simulink model "eovsa_corr_300mhz"  (R2012b)
settings: Solver=VariableStepDiscrete  SolverMode=SingleTasking  StartTime=0.0  StopTime=5000  RelTol=1e-3
undefined symbols (not defined in the file or in its folder): A, B, gcbh, PCIN, sfp, xlBlockLoadCallback, xlipgetpartsetting
libraries: xbsIndex_r4 x5996, casper_library_misc x52, simulink x33, dspsigops x24, xps_library x15, casper_library_delays x2
(part 25 of 65)

== system eovsa_corr_300mhz/swreg/pkt_fft ==
  sim_1 : Inport
  eovsa_corr_300mhz_swreg_pkt_fft_user_data_out : xbsIndex_r4/Gateway In  gui_display_data_type=Fixed-point  arith_type=Unsigned  n_bits=32  bin_pt=0  preci_type=Single  exp_width=8  frac_width=24  quantization="Round  (unbiased: +/- Inf)"  overflow=Saturate  period=1  dbl_ovrd=off  timing_constraint=None  locs_specified=off  LOCs={}  UseAsADC=off  ADCChannel='1'  inherit_from_input=off  hdl_port=on  block_type=gatewayin
  io_delay : xbsIndex_r4/Delay  rst=off  infoeditControl=Selection of Reset will increase slice count due to use of real FFs and instead of SRLs  en=off  latency=0  dbl_ovrd=off  reg_retiming=on  block_type=delay
  reint1 : xbsIndex_r4/Reinterpret  force_arith_type=on  arith_type=Unsigned  force_bin_pt=on  bin_pt=0  block_type=reinterpret
  slice_reg : xbsIndex_r4/Slice  nbits=32  boolean_output=off  mode=Lower Bit Location + Width  bit1=0  base1=MSB of Input  bit0=0  base0=LSB of Input  dbl_ovrd=off  block_type=slice
  in_reg : Outport
  wires:
  eovsa_corr_300mhz_swreg_pkt_fft_user_data_out/1 -> io_delay/1
  sim_1/1 -> eovsa_corr_300mhz_swreg_pkt_fft_user_data_out/1
  io_delay/1 -> slice_reg/1
  slice_reg/1 -> reint1/1
  reint1/1 -> in_reg/1

== system eovsa_corr_300mhz/swreg/rst ==
  sim_1 : Inport
  eovsa_corr_300mhz_swreg_rst_user_data_out : xbsIndex_r4/Gateway In  gui_display_data_type=Fixed-point  arith_type=Unsigned  n_bits=32  bin_pt=0  preci_type=Single  exp_width=8  frac_width=24  quantization="Round  (unbiased: +/- Inf)"  overflow=Saturate  period=1  dbl_ovrd=off  timing_constraint=None  locs_specified=off  LOCs={}  UseAsADC=off  ADCChannel='1'  inherit_from_input=off  hdl_port=on  block_type=gatewayin
  io_delay : xbsIndex_r4/Delay  rst=off  infoeditControl=Selection of Reset will increase slice count due to use of real FFs and instead of SRLs  en=off  latency=0  dbl_ovrd=off  reg_retiming=on  block_type=delay
  reint1 : xbsIndex_r4/Reinterpret  force_arith_type=on  arith_type=Unsigned  force_bin_pt=on  bin_pt=0  block_type=reinterpret
  slice_reg : xbsIndex_r4/Slice  nbits=32  boolean_output=off  mode=Lower Bit Location + Width  bit1=0  base1=MSB of Input  bit0=0  base0=LSB of Input  dbl_ovrd=off  block_type=slice
  in_reg : Outport
  wires:
  eovsa_corr_300mhz_swreg_rst_user_data_out/1 -> io_delay/1
  sim_1/1 -> eovsa_corr_300mhz_swreg_rst_user_data_out/1
  io_delay/1 -> slice_reg/1
  slice_reg/1 -> reint1/1
  reint1/1 -> in_reg/1

== system eovsa_corr_300mhz/swreg/snap_select ==
  sim_1 : Inport
  eovsa_corr_300mhz_swreg_snap_select_user_data_out : xbsIndex_r4/Gateway In  gui_display_data_type=Fixed-point  arith_type=Unsigned  n_bits=32  bin_pt=0  preci_type=Single  exp_width=8  frac_width=24  quantization="Round  (unbiased: +/- Inf)"  overflow=Saturate  period=1  dbl_ovrd=off  timing_constraint=None  locs_specified=off  LOCs={}  UseAsADC=off  ADCChannel='1'  inherit_from_input=off  hdl_port=on  block_type=gatewayin
  io_delay : xbsIndex_r4/Delay  rst=off  infoeditControl=Selection of Reset will increase slice count due to use of real FFs and instead of SRLs  en=off  latency=0  dbl_ovrd=off  reg_retiming=on  block_type=delay
  reint1 : xbsIndex_r4/Reinterpret  force_arith_type=on  arith_type=Unsigned  force_bin_pt=on  bin_pt=0  block_type=reinterpret
  slice_reg : xbsIndex_r4/Slice  nbits=32  boolean_output=off  mode=Lower Bit Location + Width  bit1=0  base1=MSB of Input  bit0=0  base0=LSB of Input  dbl_ovrd=off  block_type=slice
  in_reg : Outport
  wires:
  eovsa_corr_300mhz_swreg_snap_select_user_data_out/1 -> io_delay/1
  sim_1/1 -> eovsa_corr_300mhz_swreg_snap_select_user_data_out/1
  io_delay/1 -> slice_reg/1
  slice_reg/1 -> reint1/1
  reint1/1 -> in_reg/1

== system eovsa_corr_300mhz/swreg/x_op_select ==
  sim_1 : Inport
  eovsa_corr_300mhz_swreg_x_op_select_user_data_out : xbsIndex_r4/Gateway In  gui_display_data_type=Fixed-point  arith_type=Unsigned  n_bits=32  bin_pt=0  preci_type=Single  exp_width=8  frac_width=24  quantization="Round  (unbiased: +/- Inf)"  overflow=Saturate  period=1  dbl_ovrd=off  timing_constraint=None  locs_specified=off  LOCs={}  UseAsADC=off  ADCChannel='1'  inherit_from_input=off  hdl_port=on  block_type=gatewayin
  io_delay : xbsIndex_r4/Delay  rst=off  infoeditControl=Selection of Reset will increase slice count due to use of real FFs and instead of SRLs  en=off  latency=0  dbl_ovrd=off  reg_retiming=on  block_type=delay
  reint1 : xbsIndex_r4/Reinterpret  force_arith_type=on  arith_type=Unsigned  force_bin_pt=on  bin_pt=0  block_type=reinterpret
  slice_reg : xbsIndex_r4/Slice  nbits=32  boolean_output=off  mode=Lower Bit Location + Width  bit1=0  base1=MSB of Input  bit0=0  base0=LSB of Input  dbl_ovrd=off  block_type=slice
  in_reg : Outport
  wires:
  eovsa_corr_300mhz_swreg_x_op_select_user_data_out/1 -> io_delay/1
  sim_1/1 -> eovsa_corr_300mhz_swreg_x_op_select_user_data_out/1
  io_delay/1 -> slice_reg/1
  slice_reg/1 -> reint1/1
  reint1/1 -> in_reg/1

== system eovsa_corr_300mhz/timing/arm_sync ==
  arm : Inport
  pps_in : Inport  Port=2
  data_in : Inport  Port=3
  adc0_over : Inport  Port=4
  adc1_over : Inport  Port=5
  Delay1 : xbsIndex_r4/Delay  rst=off  infoeditControl=Selection of Reset will increase slice count due to use of real FFs and instead of SRLs  en=on  latency=1  dbl_ovrd=off  reg_retiming=on  block_type=delay
      settings: block_version=11.4
  Delay13 : xbsIndex_r4/Delay  rst=off  infoeditControl=Selection of Reset will increase slice count due to use of real FFs and instead of SRLs  en=on  latency=1  dbl_ovrd=off  reg_retiming=on  block_type=delay
      settings: block_version=11.4
  Delay2 : xbsIndex_r4/Delay  rst=off  infoeditControl=Selection of Reset will increase slice count due to use of real FFs and instead of SRLs  en=on  latency=1  dbl_ovrd=off  reg_retiming=on  block_type=delay
      settings: block_version=11.4
  Delay{3..6} (4 alike) : xbsIndex_r4/Delay  rst=off  infoeditControl=Selection of Reset will increase slice count due to use of real FFs and instead of SRLs  en=off  latency=1  dbl_ovrd=off  reg_retiming=on  block_type=delay
      settings: block_version=11.4
  Logical12 : xbsIndex_r4/Logical  logical_function=AND  inputs=2  en=off  latency=0  precision=Full  arith_type=Unsigned  n_bits=16  bin_pt=0  align_bp=on  dbl_ovrd=off  block_type=logical
      settings: block_version=11.4
  Logical3 : xbsIndex_r4/Logical  logical_function=AND  inputs=2  en=off  latency=0  precision=Full  arith_type=Unsigned  n_bits=16  bin_pt=0  align_bp=on  dbl_ovrd=off  block_type=logical
      settings: block_version=11.4
  Logical4 : xbsIndex_r4/Logical  logical_function=OR  inputs=2  en=off  latency=1  precision=Full  arith_type=Unsigned  n_bits=16  bin_pt=0  align_bp=on  dbl_ovrd=off  block_type=logical
      settings: block_version=11.4
  edge_detect : Subsystem  AncestorBlock=casper_library_misc/edge_detect  mask(edge_detect){edge=Rising, polarity=Active High, x_in=[0 0.08 0.08 0.16 0.16 0.24 0.24 0.32 0.32 0.4], y_in=[-1 -1  1  1  1  1  1  1  1  1], x_out=[0.6 0.68 0.68 0.76 0.76 0.84 0.84 0.92 0.92 1], y_out=[-1 -1  1  1 -1 -1 -1 -1 -1 -1]}
      mask prompts: edge "Edge Type"; polarity "Output Polarity"; x_in "Input X Positions"; y_in "Input Y Positions"; x_out "Output X Positions"; y_out "Output Y Positions"
      mask help: Output is active for one-cycle after each edge of the specified type (i.e. rising, falling or both).
      mask init: same as eovsa_corr_300mhz/edge_detect1
      settings: AttributesFormatString=|
      | rising edges
      | active high
      mask Help: Output is active for one-cycle after each edge of the specified type (i.e. rising, falling, or both).  Latency is zero.
      mask TypeOptions edge: Rising | Falling | Both
      mask TypeOptions polarity: Active High | Active Low
      mask Display:
      | plot(x_in_num,0.5+y_in_num*0.2);
      | plot(x_out_num,0.5+y_out_num*0.2);
  edge_detect1 : Subsystem  AncestorBlock=casper_library_misc/edge_detect  mask(edge_detect){edge=Rising, polarity=Active High, x_in=[0 0.08 0.08 0.16 0.16 0.24 0.24 0.32 0.32 0.4], y_in=[-1 -1  1  1  1  1  1  1  1  1], x_out=[0.6 0.68 0.68 0.76 0.76 0.84 0.84 0.92 0.92 1], y_out=[-1 -1  1  1 -1 -1 -1 -1 -1 -1]}
      mask prompts: edge "Edge Type"; polarity "Output Polarity"; x_in "Input X Positions"; y_in "Input Y Positions"; x_out "Output X Positions"; y_out "Output Y Positions"
      mask help: Output is active for one-cycle after each edge of the specified type (i.e. rising, falling or both).
      mask init: same as eovsa_corr_300mhz/edge_detect1
      settings: AttributesFormatString=|
      | rising edges
      | active high
      mask Help: Output is active for one-cycle after each edge of the specified type (i.e. rising, falling, or both).  Latency is zero.
      mask TypeOptions edge: Rising | Falling | Both
      mask TypeOptions polarity: Active High | Active Low
      mask Display:
      | plot(x_in_num,0.5+y_in_num*0.2);
      | plot(x_out_num,0.5+y_out_num*0.2);
  sync : Outport
  data_out : Outport  Port=2
  pps : Outport  Port=3
  armed : Outport  Port=4
  synced : Outport  Port=5
  adc_overflow : Outport  Port=6
  wires:
  arm/1 -> edge_detect/1(in)
  Logical12/1 -> Delay13/1, Delay13/2
  pps_in/1 -> Logical12/2, Logical3/2
  edge_detect/1(out) -> Delay1/1, Delay1/2
  Delay1/1 -> Logical12/1, armed/1
  Delay13/1 -> Logical3/1
  data_in/1 -> Delay4/1
  Delay4/1 -> Delay3/1
  Logical3/1 -> Delay2/1, Delay2/2, Delay5/1
  Delay2/1 -> edge_detect1/1(in), synced/1
  edge_detect1/1(out) -> sync/1
  Delay3/1 -> data_out/1
  Delay5/1 -> pps/1
  adc0_over/1 -> Logical4/1
  adc1_over/1 -> Logical4/2
  Logical4/1 -> Delay6/1
  Delay6/1 -> adc_overflow/1

== system eovsa_corr_300mhz/tx_pkt/add_gen ==
  note: To storage
  note: prevent one extra
      | write to address 0
  note: Do one
      | capture by
      | default
  note: Count of bytes in BRAM
      | as well as done signal
  note: A total count of
      | bytes written to
      | BRAM since trig
  note: Force MSbit of count
      | to be '1' by negating busy
      | as counter bit may be '0' or '1'
  vin : Inport
  din : Inport  Port=2
  we : Inport  Port=3
  go : Inport  Port=4
  cont : Inport  Port=5
  init : Inport  Port=6
  Concat : xbsIndex_r4/Concat  num_inputs=3  dbl_ovrd=off  block_type=concat
      settings: block_version=10.1.3
  Convert : xbsIndex_r4/Convert  gui_display_data_type=Fixed-point  arith_type=Unsigned  n_bits=32-nsamples-log2(increment)-1  bin_pt=0  float_type=Single  exp_bits=8  fraction_bits=24  quantization=Truncate  overflow=Wrap  en=off  latency=0  dbl_ovrd=off  pipeline=off  block_type=convert
      settings: block_version=10.1.3
  Delay{,1..7} (8 alike) : xbsIndex_r4/Delay  rst=off  infoeditControl=Selection of Reset will increase slice count due to use of real FFs and instead of SRLs  en=off  latency=1  dbl_ovrd=off  reg_retiming=on  block_type=delay
      settings: block_version=11.4
  Inverter : xbsIndex_r4/Inverter  en=off  latency=1  dbl_ovrd=off  block_type=inv
      settings: block_version=11.4
  Inverter1 : xbsIndex_r4/Inverter  en=off  latency=0  dbl_ovrd=off  block_type=inv
      settings: block_version=11.4
  Logical1 : xbsIndex_r4/Logical  logical_function=AND  inputs=2  en=off  latency=1  precision=Full  arith_type=Unsigned  n_bits=8  bin_pt=2  align_bp=on  dbl_ovrd=off  block_type=logical
      settings: xl_area=[0, 0, 0, 0, 0, 0, 0]
  Logical2 : xbsIndex_r4/Logical  logical_function=AND  inputs=2  en=off  latency=1  precision=Full  arith_type=Unsigned  n_bits=8  bin_pt=2  align_bp=on  dbl_ovrd=off  block_type=logical
      settings: xl_area=[0, 0, 0, 0, 0, 0, 0]
  Logical4 : xbsIndex_r4/Logical  logical_function=OR  inputs=2  en=off  latency=0  precision=Full  arith_type=Unsigned  n_bits=8  bin_pt=2  align_bp=on  dbl_ovrd=off  block_type=logical
      settings: xl_area=[0, 0, 0, 0, 0, 0, 0]
  Logical6 : xbsIndex_r4/Logical  logical_function=AND  inputs=3  en=off  latency=0  precision=Full  arith_type=Unsigned  n_bits=8  bin_pt=2  align_bp=on  dbl_ovrd=off  block_type=logical
      settings: xl_area=[0, 0, 0, 0, 0, 0, 0]
  Register3 : xbsIndex_r4/Register  init=0  rst=on  en=on  dbl_ovrd=off  block_type=register
      settings: xl_area=[0, 0, 0, 0, 0, 0, 0]
  Register4 : xbsIndex_r4/Register  init=0  rst=off  en=on  dbl_ovrd=off  block_type=register
      settings: xl_area=[0, 0, 0, 0, 0, 0, 0]
  Register5 : xbsIndex_r4/Register  init=1  rst=on  en=on  dbl_ovrd=off  block_type=register
      settings: xl_area=[0, 0, 0, 0, 0, 0, 0]
  Shift : xbsIndex_r4/Shift  shift_dir=Left  shift_bits=32-nsamples-log2(increment)-1-1  en=off  latency=1  precision=Full  arith_type="Signed  (2's comp)"  n_bits=16  bin_pt=14  quantization=Truncate  overflow=Wrap  dbl_ovrd=off  block_type=shift
  add_gen : xbsIndex_r4/Counter  cnt_type=Free Running  cnt_to=1  operation=Up  start_count=0  cnt_by_val=increment  arith_type=Unsigned  n_bits=counter_size  bin_pt=0  load_pin=off  rst=on  en=on  explicit_period=on  period=1  dbl_ovrd=off  use_behavioral_HDL=off  implementation=DSP48  use_rpm=on  block_type=counter
      settings: xl_area=[0, 0, 0, 0, 0, 0, 0]
  edge_detect : Subsystem  AncestorBlock=casper_library_misc/edge_detect  mask(edge_detect){edge=Both, polarity=Active High, x_in=[0 0.08 0.08 0.16 0.16 0.24 0.24 0.32 0.32 0.4], y_in=[-1 -1  1  1  1  1 -1 -1 -1 -1], x_out=[0.6 0.68 0.68 0.76 0.76 0.84 0.84 0.92 0.92 1], y_out=[-1 -1  1  1 -1 -1  1  1 -1 -1]}
      mask prompts: edge "Edge Type"; polarity "Output Polarity"; x_in "Input X Positions"; y_in "Input Y Positions"; x_out "Output X Positions"; y_out "Output Y Positions"
      mask help: Output is active for one-cycle after each edge of the specified type (i.e. rising, falling or both).
      mask init: same as eovsa_corr_300mhz/edge_detect1
      settings: AttributesFormatString=|
      | both edges
      | active high
      mask Help: Output is active for one-cycle after each edge of the specified type (i.e. rising, falling, or both).  Latency is zero.
      mask TypeOptions edge: Rising | Falling | Both
      mask TypeOptions polarity: Active High | Active Low
      mask Display:
      | plot(x_in_num,0.5+y_in_num*0.2);
      | plot(x_out_num,0.5+y_out_num*0.2);
  slice1 : xbsIndex_r4/Slice  nbits=nsamples+log2(increment)  boolean_output=off  mode=Lower Bit Location + Width  bit1=0  base1=LSB of Input  bit0=0  base0=LSB of Input  dbl_ovrd=off  block_type=slice
      settings: block_version=10.1.3
  slice2 : xbsIndex_r4/Slice  nbits=nsamples-burst_size  boolean_output=off  mode=Lower Bit Location + Width  bit1=0  base1=LSB of Input  bit0=log2(increment)+burst_size  base0=LSB of Input  dbl_ovrd=off  block_type=slice
      settings: block_version=10.1.3
  slice3 : xbsIndex_r4/Slice  nbits=1  boolean_output=on  mode=Lower Bit Location + Width  bit1=0  base1=MSB of Input  bit0=nsamples + log2(increment)  base0=LSB of Input  dbl_ovrd=off  block_type=slice
      settings: block_version=10.1.3
  vout : Outport
  add : Outport  Port=2
  dout : Outport  Port=3
  we_o : Outport  Port=4
  status : Outport  Port=5
  en_cnt : Outport  Port=6
  wires:
  Shift/1 -> Concat/1
  Delay/1 -> Register5/2
  Inverter1/1 -> Logical4/2
  cont/1 -> Delay3/1
  edge_detect/1(out) -> Inverter1/1, Register5/3
  Register4/1 -> vout/1
  Logical2/1 -> Register4/2
  Register3/1 -> Logical2/2
  vin/1 -> Delay5/1
  add_gen/1 -> slice2/1, slice1/1, Delay2/1, slice3/1
  Register5/1 -> Convert/1, Inverter/1, Logical6/1
  slice3/1 -> edge_detect/1(in)
  init/1 -> Delay4/1
  Logical6/1 -> we_o/1, Logical2/1, Register3/2, add_gen/2
  Concat/1 -> status/1
  Convert/1 -> Shift/1
  slice2/1 -> add/1
  Delay2/1 -> en_cnt/1
  din/1 -> Delay6/1
  Delay1/1 -> Concat/3
  slice1/1 -> Delay1/1
  Inverter/1 -> Concat/2
  Logical4/1 -> Logical6/2
  we/1 -> Logical1/1
  go/1 -> Logical1/2
  Logical1/1 -> Logical6/3
  Delay7/1 -> Register4/1
  Delay3/1 -> Logical4/1, Register5/1
  Delay4/1 -> Register3/3, Register3/1, add_gen/1, Delay/1
  Delay5/1 -> Delay7/1
  Delay6/1 -> dout/1

== system eovsa_corr_300mhz/tx_pkt/basic_ctrl ==
  vin : Inport
  din : Inport  Port=2
  we : Inport  Port=3
  trig : Inport  Port=4
  ctrl : Inport  Port=5
  stopi : Inport  Port=6
  Constant : xbsIndex_r4/Constant  const=1  gui_display_data_type=Fixed-point  arith_type=Boolean  n_bits=16  bin_pt=14  preci_type=Single  exp_width=8  frac_width=24  explicit_period=on  period=1  equ=P=C  opselect=C  inp2=PCIN>>17  opr=+  inp1=P  carry=CIN  dbl_ovrd=off  block_type=constant
      settings: block_version=11.4
  Constant1 : xbsIndex_r4/Constant  const=1  gui_display_data_type=Fixed-point  arith_type=Boolean  n_bits=1  bin_pt=0  preci_type=Single  exp_width=8  frac_width=24  explicit_period=on  period=1  equ=P=C  opselect=C  inp2=PCIN>>17  opr=+  inp1=P  carry=CIN  dbl_ovrd=off  block_type=constant
  Constant2 : xbsIndex_r4/Constant  const=1  gui_display_data_type=Fixed-point  arith_type=Boolean  n_bits=1  bin_pt=0  preci_type=Single  exp_width=8  frac_width=24  explicit_period=on  period=1  equ=P=C  opselect=C  inp2=PCIN>>17  opr=+  inp1=P  carry=CIN  dbl_ovrd=off  block_type=constant
  Delay1 : xbsIndex_r4/Delay  rst=off  infoeditControl=Selection of Reset will increase slice count due to use of real FFs and instead of SRLs  en=off  latency=1  dbl_ovrd=off  reg_retiming=on  block_type=delay
      settings: block_version=11.4
  Delay2 : xbsIndex_r4/Delay  rst=off  infoeditControl=Selection of Reset will increase slice count due to use of real FFs and instead of SRLs  en=off  latency=1  dbl_ovrd=off  reg_retiming=on  block_type=delay
      settings: block_version=11.4
  Delay3 : xbsIndex_r4/Delay  rst=off  infoeditControl=Selection of Reset will increase slice count due to use of real FFs and instead of SRLs  en=off  latency=1  dbl_ovrd=off  reg_retiming=on  block_type=delay
      settings: block_version=11.4
  Inverter : xbsIndex_r4/Inverter  en=off  latency=0  dbl_ovrd=off  block_type=inv
      settings: block_version=11.4
  Logical : xbsIndex_r4/Logical  logical_function=AND  inputs=2  en=off  latency=0  precision=Full  arith_type=Unsigned  n_bits=16  bin_pt=0  align_bp=on  dbl_ovrd=off  block_type=logical
      settings: block_version=11.4
  Mux1 : xbsIndex_r4/Mux  inputs=2  en=off  latency=0  precision=Full  arith_type="Signed  (2's comp)"  n_bits=8  bin_pt=2  quantization=Truncate  overflow=Wrap  dbl_ovrd=off  block_type=mux
      settings: xl_area=[0, 0, 0, 0, 0, 0, 0]
  Mux2 : xbsIndex_r4/Mux  inputs=2  en=off  latency=0  precision=Full  arith_type="Signed  (2's comp)"  n_bits=8  bin_pt=2  quantization=Truncate  overflow=Wrap  dbl_ovrd=off  block_type=mux
      settings: xl_area=[0, 0, 0, 0, 0, 0, 0]
  Register1 : xbsIndex_r4/Register  init=0  rst=on  en=on  dbl_ovrd=off  block_type=register
      settings: xl_area=[0, 0, 0, 0, 0, 0, 0]
  Register6 : xbsIndex_r4/Register  init=0  rst=on  en=on  dbl_ovrd=off  block_type=register
      settings: xl_area=[0, 0, 0, 0, 0, 0, 0]
  dram_munge : Subsystem  mask{dram=off, data_width=data_width}
      mask prompts: data_width "data width"
      mask init: same as eovsa_corr_300mhz/rx_hdr/basic_ctrl/dram_munge
  edge_detect : casper_library_misc/edge_detect  edge=Rising  polarity=Active High  x_in=[0 0.08 0.08 0.16 0.16 0.24 0.24 0.32 0.32 0.4]  y_in="[-1 -1  1  1  1  1  1  1  1  1]"  x_out=[0.6 0.68 0.68 0.76 0.76 0.84 0.84 0.92 0.92 1]  y_out="[-1 -1  1  1 -1 -1 -1 -1 -1 -1]"
  enable : xbsIndex_r4/Slice  nbits=1  boolean_output=on  mode=Lower Bit Location + Width  bit1=0  base1=LSB of Input  bit0=0  base0=LSB of Input  dbl_ovrd=off  block_type=slice
      settings: infoedit="Extracts a given range of bits from each input sample and presents it at the output.  The output type is ordinarily unsigned with binary point at zero, but can be Boolean when the slice is one bit wide.<P><P>Hardware notes: In hardware this block costs nothing."  block_version=10.1.3
  trig_src : xbsIndex_r4/Slice  nbits=1  boolean_output=on  mode=Lower Bit Location + Width  bit1=0  base1=LSB of Input  bit0=1  base0=LSB of Input  dbl_ovrd=off  block_type=slice
      settings: infoedit="Extracts a given range of bits from each input sample and presents it at the output.  The output type is ordinarily unsigned with binary point at zero, but can be Boolean when the slice is one bit wide.<P><P>Hardware notes: In hardware this block costs nothing."  block_version=10.1.3
  valid_src : xbsIndex_r4/Slice  nbits=1  boolean_output=on  mode=Lower Bit Location + Width  bit1=0  base1=LSB of Input  bit0=2  base0=LSB of Input  dbl_ovrd=off  block_type=slice
      settings: infoedit="Extracts a given range of bits from each input sample and presents it at the output.  The output type is ordinarily unsigned with binary point at zero, but can be Boolean when the slice is one bit wide.<P><P>Hardware notes: In hardware this block costs nothing."  block_version=10.1.3
  vout : Outport
  dout : Outport  Port=2
  we_o : Outport  Port=3
  go : Outport  Port=4
  stop : Outport  Port=5
  init : Outport  Port=6
  wires:
  Delay1/1 -> edge_detect/1
  Delay3/1 -> Mux1/1
  Delay2/1 -> Mux2/1
  dram_munge/1(vout) -> vout/1
  vin/1 -> dram_munge/1(vin)
  dram_munge/3(we_o) -> we_o/1
  dram_munge/2(dout) -> dout/1
  din/1 -> dram_munge/2(din)
  Inverter/1 -> Logical/2
  Mux2/1 -> Logical/1, Register6/1
  Register6/1 -> go/1
  trig/1 -> Mux2/2
  Mux1/1 -> dram_munge/3(we)
  we/1 -> Mux1/2
  ctrl/1 -> enable/1, valid_src/1, trig_src/1
  edge_detect/1 -> Inverter/1, Register1/3, dram_munge/4(init), Register6/2, init/1
  enable/1 -> Delay1/1
  Constant1/1 -> Mux2/3
  Constant2/1 -> Mux1/3
  trig_src/1 -> Delay2/1
  valid_src/1 -> Delay3/1
  Constant/1 -> Register1/1
  Register1/1 -> Register6/3
  Logical/1 -> Register1/2
  stopi/1 -> stop/1

== system eovsa_corr_300mhz/tx_pkt/bram ==
  addr : Inport
  data_in : Inport  Port=2
  we : Inport  Port=3
  calc_add : Subsystem  mask{data_width=64, addr_width=10, sample_rate=sample_rate}
      mask prompts: data_width "data width"; addr_width "address width"; sample_rate "sample rate"
  convert_addr : xbsIndex_r4/Convert  gui_display_data_type=Fixed-point  arith_type=Unsigned  n_bits=addr_width  bin_pt=0  float_type=Single  exp_bits=8  fraction_bits=24  quantization=Truncate  overflow=Wrap  en=off  latency=0  dbl_ovrd=off  pipeline=off  block_type=convert
      settings: xl_area=[0, 0, 0, 0, 0, 0, 0]
  convert_din1 : xbsIndex_r4/Convert  gui_display_data_type=Fixed-point  arith_type=Unsigned  n_bits=64  bin_pt=0  float_type=Single  exp_bits=8  fraction_bits=24  quantization=Truncate  overflow=Wrap  en=off  latency=0  dbl_ovrd=off  pipeline=off  block_type=convert
      settings: xl_area=[0, 0, 0, 0, 0, 0, 0]
  convert_we : xbsIndex_r4/Convert  gui_display_data_type=Fixed-point  arith_type=Unsigned  n_bits=1  bin_pt=0  float_type=Single  exp_bits=8  fraction_bits=24  quantization=Truncate  overflow=Wrap  en=off  latency=0  dbl_ovrd=off  pipeline=off  block_type=convert
      settings: xl_area=[0, 0, 0, 0, 0, 0, 0]
  eovsa_corr_300mhz_tx_pkt_bram_addr : xbsIndex_r4/Gateway Out  inherit_from_input=off  hdl_port=on  timing_constraint=None  locs_specified=off  LOCs={'A5','B9','A9','C1','A3','G6','E9','A6','A7','A8','B8','B1','B3','D9','B5','B4','B6','C2'}  UseAsDAC=off  DACChannel='1'  block_type=gatewayout
      settings: infoedit="Gateway out block.  Converts Xilinx fixed point inputs into ouputs of type Simulink integer, double, or fixed point.<P><P>Hardware notes:  In hardware these blocks become top level output ports or are discarded, depending on how they are configured."  xl_area=[0, 0, 0, 0, 0, 0, 0]  sginterface={'Nallatech'=>{'xdspkit'=>{'non_memory_mapped_port'=>'uprev_Shared_BRAM_addr'}},'Xilinx'=>{'jtaghwcosim'=>{'non_memory_mapped_port'=>'uprev_Shared_BRAM_addr'},'xdspkit'=>{'non_memory_mapped_port'=>'uprev_Shared_BRAM_addr'}}}
  eovsa_corr_300mhz_tx_pkt_bram_data_in : xbsIndex_r4/Gateway Out  inherit_from_input=off  hdl_port=on  timing_constraint=None  locs_specified=off  LOCs={'B21','B22','A22','B23','B19','C19','A20','A21','A23','B24','A24','A25','E18','D18','C18','B18'}  UseAsDAC=off  DACChannel='1'  block_type=gatewayout
      settings: infoedit="Gateway out block.  Converts Xilinx fixed point inputs into ouputs of type Simulink integer, double, or fixed point.<P><P>Hardware notes:  In hardware these blocks become top level output ports or are discarded, depending on how they are configured."  xl_area=[0, 0, 0, 0, 0, 0, 0]  sginterface={'Nallatech'=>{'xdspkit'=>{'non_memory_mapped_port'=>'uprev_Shared_BRAM_data_in'}},'Xilinx'=>{'jtaghwcosim'=>{'non_memory_mapped_port'=>'uprev_Shared_BRAM_data_in'},'xdspkit'=>{'non_memory_mapped_port'=>'uprev_Shared_BRAM_data_in'}}}
  eovsa_corr_300mhz_tx_pkt_bram_data_out : xbsIndex_r4/Gateway In  gui_display_data_type=Fixed-point  arith_type=Unsigned  n_bits=64  bin_pt=0  preci_type=Single  exp_width=8  frac_width=24  quantization=Truncate  overflow=Wrap  period=sample_rate  dbl_ovrd=off  timing_constraint=None  locs_specified=off  LOCs={}  UseAsADC=off  ADCChannel='1'  inherit_from_input=off  hdl_port=on  block_type=gatewayin
      settings: xl_area=[0, 0, 0, 0, 0, 0, 0]
  eovsa_corr_300mhz_tx_pkt_bram_we : xbsIndex_r4/Gateway Out  inherit_from_input=off  hdl_port=on  timing_constraint=None  locs_specified=off  LOCs={'A14'}  UseAsDAC=off  DACChannel='1'  block_type=gatewayout
      settings: infoedit="Gateway out block.  Converts Xilinx fixed point inputs into ouputs of type Simulink integer, double, or fixed point.<P><P>Hardware notes:  In hardware these blocks become top level output ports or are discarded, depending on how they are configured."  xl_area=[0, 0, 0, 0, 0, 0, 0]
  mem : Subsystem
  munge_in : Subsystem  AncestorBlock=casper_library_flow_control/munge  mask(munge){divisions=2, div_size=[32 32], order=[1  0], arith_type_out=Unsigned, bin_pt_out=0}
      mask prompts: divisions "Number of divisions"; div_size "Division size (bits)"; order "Division packing order"; arith_type_out "Output arithmetic type"; bin_pt_out "Output binary point"
      mask help: Splits an input bus into the specified number of divisions and then recombines them in the order specified (most significant division = 0,least = number divisions-1)
      mask init:
      | munge_init(gcb, ...
      |     'divisions', divisions, ...
      |     'div_size', div_size, ...
      |     'order', order, ...
      |     'arith_type_out', arith_type_out, ...
      |     'bin_pt_out', bin_pt_out);
      settings: AttributesFormatString=|
      | split:[32 32]
      | join:[1 0]
      | Unsigned [64,0]
      mask TypeOptions arith_type_out: Unsigned | Signed  (2's comp) | Floating-point
  munge_out : Subsystem  AncestorBlock=casper_library_flow_control/munge  mask(munge){divisions=2, div_size=[32 32], order=[1  0], arith_type_out=Unsigned, bin_pt_out=0}
      mask prompts: divisions "Number of divisions"; div_size "Division size (bits)"; order "Division packing order"; arith_type_out "Output arithmetic type"; bin_pt_out "Output binary point"
      mask help: Splits an input bus into the specified number of divisions and then recombines them in the order specified (most significant division = 0,least = number divisions-1)
      mask init:
      | munge_init(gcb, ...
      |     'divisions', divisions, ...
      |     'div_size', div_size, ...
      |     'order', order, ...
      |     'arith_type_out', arith_type_out, ...
      |     'bin_pt_out', bin_pt_out);
      settings: AttributesFormatString=|
      | split:[32 32]
      | join:[1 0]
      | Unsigned [64,0]
      mask TypeOptions arith_type_out: Unsigned | Signed  (2's comp) | Floating-point
  data_out : Outport
  wires:
  munge_in/1(dout) -> convert_din1/1
  munge_out/1(dout) -> data_out/1
  we/1 -> convert_we/1
  addr/1 -> calc_add/1(in)
  mem/1(Out1) -> eovsa_corr_300mhz_tx_pkt_bram_data_out/1
  eovsa_corr_300mhz_tx_pkt_bram_data_out/1 -> munge_out/1(din)
  convert_we/1 -> eovsa_corr_300mhz_tx_pkt_bram_we/1
  eovsa_corr_300mhz_tx_pkt_bram_addr/1 -> mem/1(In1)
  eovsa_corr_300mhz_tx_pkt_bram_data_in/1 -> mem/2(In2)
  eovsa_corr_300mhz_tx_pkt_bram_we/1 -> mem/3(In3)
  calc_add/1(out) -> convert_addr/1
  data_in/1 -> munge_in/1(din)
  convert_din1/1 -> eovsa_corr_300mhz_tx_pkt_bram_data_in/1
  convert_addr/1 -> eovsa_corr_300mhz_tx_pkt_bram_addr/1

== system eovsa_corr_300mhz/tx_pkt/ctrl ==
  sim_1 : Inport
  eovsa_corr_300mhz_tx_pkt_ctrl_user_data_out : xbsIndex_r4/Gateway In  gui_display_data_type=Fixed-point  arith_type=Unsigned  n_bits=32  bin_pt=0  preci_type=Single  exp_width=8  frac_width=24  quantization="Round  (unbiased: +/- Inf)"  overflow=Saturate  period=1  dbl_ovrd=off  timing_constraint=None  locs_specified=off  LOCs={}  UseAsADC=off  ADCChannel='1'  inherit_from_input=off  hdl_port=on  block_type=gatewayin
  io_delay : xbsIndex_r4/Delay  rst=off  infoeditControl=Selection of Reset will increase slice count due to use of real FFs and instead of SRLs  en=off  latency=0  dbl_ovrd=off  reg_retiming=on  block_type=delay
  reint1 : xbsIndex_r4/Reinterpret  force_arith_type=on  arith_type=Unsigned  force_bin_pt=on  bin_pt=0  block_type=reinterpret
  slice_reg : xbsIndex_r4/Slice  nbits=32  boolean_output=off  mode=Lower Bit Location + Width  bit1=0  base1=MSB of Input  bit0=0  base0=LSB of Input  dbl_ovrd=off  block_type=slice
  in_reg : Outport
  wires:
  eovsa_corr_300mhz_tx_pkt_ctrl_user_data_out/1 -> io_delay/1
  sim_1/1 -> eovsa_corr_300mhz_tx_pkt_ctrl_user_data_out/1
  io_delay/1 -> slice_reg/1
  slice_reg/1 -> reint1/1
  reint1/1 -> in_reg/1

== system eovsa_corr_300mhz/tx_pkt/status ==
  out_reg : Inport
  assert_reg : xbsIndex_r4/Assert  assert_type=on  type_source=Explicitly  gui_display_data_type=Fixed-point  arith_type=Unsigned  n_bits=32  bin_pt=0  preci_type=Single  exp_width=8  frac_width=24  assert_rate=off  rate_source=Explicitly  period=1  output_port=on  block_type=assert
  cast_gw : xbsIndex_r4/Convert  gui_display_data_type=Fixed-point  arith_type=Unsigned  n_bits=32  bin_pt=0  float_type=Single  exp_bits=8  fraction_bits=24  quantization=Truncate  overflow=Wrap  en=off  latency=0  dbl_ovrd=off  pipeline=off  block_type=convert
  eovsa_corr_300mhz_tx_pkt_status_user_data_in : xbsIndex_r4/Gateway Out  inherit_from_input=off  hdl_port=on  timing_constraint=None  locs_specified=off  LOCs={}  UseAsDAC=off  DACChannel='1'  block_type=gatewayout
  io_delay : xbsIndex_r4/Delay  rst=off  infoeditControl=Selection of Reset will increase slice count due to use of real FFs and instead of SRLs  en=off  latency=0  dbl_ovrd=off  reg_retiming=on  block_type=delay
  reint1 : xbsIndex_r4/Reinterpret  force_arith_type=on  arith_type=Unsigned  force_bin_pt=on  bin_pt=0  block_type=reinterpret
  sim_out : Outport
  wires:
  io_delay/1 -> cast_gw/1
  cast_gw/1 -> eovsa_corr_300mhz_tx_pkt_status_user_data_in/1
  eovsa_corr_300mhz_tx_pkt_status_user_data_in/1 -> sim_out/1
  out_reg/1 -> assert_reg/1
  assert_reg/1 -> reint1/1
  reint1/1 -> io_delay/1

== system eovsa_corr_300mhz/vector_acc/edge_detect ==
  in : Inport
  Delay : xbsIndex_r4/Delay  rst=off  infoeditControl=Selection of Reset will increase slice count due to use of real FFs and instead of SRLs  en=off  latency=1  dbl_ovrd=off  reg_retiming=on  block_type=delay
      settings: xl_area=[0, 0, 0, 0, 0, 0, 0]
  Inverter : xbsIndex_r4/Inverter  en=off  latency=0  dbl_ovrd=off  block_type=inv
      settings: xl_area=[0, 0, 0, 0, 0, 0, 0]
  edge_op : xbsIndex_r4/Logical  logical_function=NOR  inputs=2  en=off  latency=0  precision=Full  arith_type=Unsigned  n_bits=8  bin_pt=2  align_bp=on  dbl_ovrd=off  block_type=logical
      settings: xl_area=[0, 0, 0, 0, 0, 0, 0]
  out : Outport
  wires:
  Inverter/1 -> edge_op/1
  edge_op/1 -> out/1
  in/1 -> Inverter/1, Delay/1
  Delay/1 -> edge_op/2

== system eovsa_corr_300mhz/vector_acc/edge_detect1 ==
  in : Inport
  Delay : xbsIndex_r4/Delay  rst=off  infoeditControl=Selection of Reset will increase slice count due to use of real FFs and instead of SRLs  en=off  latency=1  dbl_ovrd=off  reg_retiming=on  block_type=delay
      settings: xl_area=[0, 0, 0, 0, 0, 0, 0]
  Inverter : xbsIndex_r4/Inverter  en=off  latency=0  dbl_ovrd=off  block_type=inv
      settings: xl_area=[0, 0, 0, 0, 0, 0, 0]
  edge_op : xbsIndex_r4/Logical  logical_function=AND  inputs=2  en=off  latency=0  precision=Full  arith_type=Unsigned  n_bits=8  bin_pt=2  align_bp=on  dbl_ovrd=off  block_type=logical
      settings: xl_area=[0, 0, 0, 0, 0, 0, 0]
  out : Outport
  wires:
  Inverter/1 -> edge_op/1
  edge_op/1 -> out/1
  in/1 -> Inverter/1, Delay/1
  Delay/1 -> edge_op/2

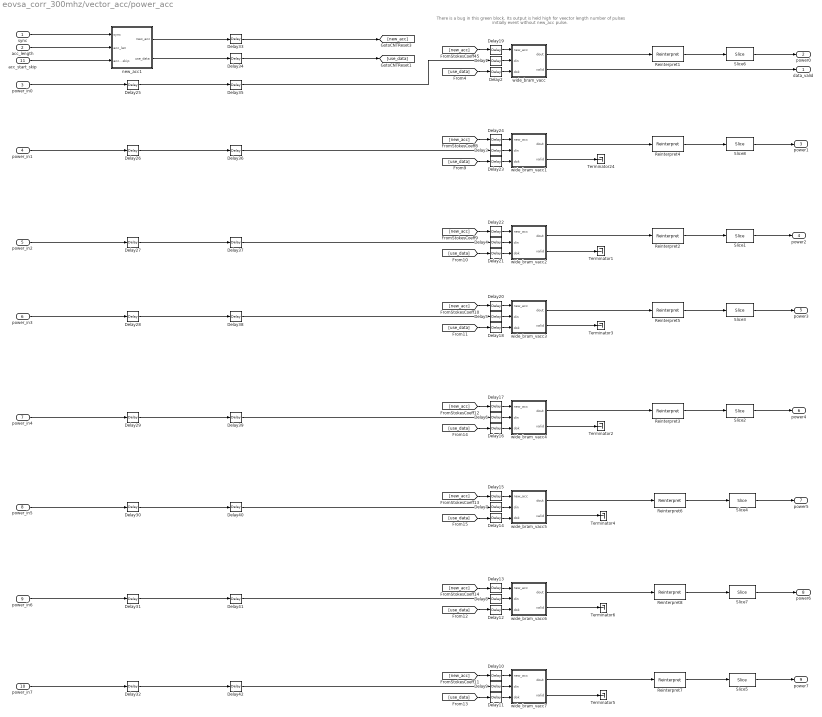
== system eovsa_corr_300mhz/vector_acc/power_acc ==
  note: There is a bug in this green block.
      | Its output is held high for veector length number of pulses initially event without new_acc pulse.
  sync : Inport
  acc_length : Inport  Port=2
  power_in0 : Inport  Port=3
  power_in1 : Inport  Port=4
  power_in2 : Inport  Port=5
  power_in3 : Inport  Port=6
  power_in4 : Inport  Port=7
  power_in5 : Inport  Port=8
  power_in6 : Inport  Port=9
  power_in7 : Inport  Port=10
  acc_start_skip : Inport  Port=11
  Delay{1,3..9,25..32,35..42} (24 alike) : xbsIndex_r4/Delay  rst=off  infoeditControl=Selection of Reset will increase slice count due to use of real FFs and instead of SRLs  en=off  latency=1  dbl_ovrd=off  reg_retiming=on  block_type=delay
      settings: block_version=11.4
  Delay{2,10..24,33..34} (18 alike) : xbsIndex_r4/Delay  rst=off  infoeditControl=Selection of Reset will increase slice count due to use of real FFs and instead of SRLs  en=off  latency=1  dbl_ovrd=off  reg_retiming=off  block_type=delay
      settings: block_version=11.4
  Reinterpret{1..8} (8 alike) : xbsIndex_r4/Reinterpret  force_arith_type=on  arith_type=Unsigned  force_bin_pt=on  bin_pt=0  block_type=reinterpret
      settings: infoedit="Changes signal type without altering the binary representation.   You can changed the signal between signed and unsigned, and relocate the binary point.<br><br>Hardware notes: In hardware this block costs nothing.<br><br>Example:  Suppose the input is 6 bits wide, signed, with 2 fractional bits, and the output is forced to unsigned with 0 fractional bits.  Then an input of -2.0 (1110.00 in binary 2's complement) becomes an output of 56 (111000 in binary)."
  Slice{1..8} (8 alike) : xbsIndex_r4/Slice  nbits=32  boolean_output=off  mode=Upper Bit Location + Width  bit1=0  base1=MSB of Input  bit0=0  base0=LSB of Input  dbl_ovrd=off  block_type=slice
  Terminator{1..6,24} (7 alike) : Terminator
  new_acc1 : Subsystem
  wide_bram_vacc : Subsystem  AncestorBlock=casper_library_accumulators/wide_bram_vacc  mask(wide_bram_vacc){vec_len=2048, arith_type=Unsigned, n_bits=52, bin_pt=34}
      mask prompts: vec_len "Vector length:"; arith_type "Arithmetic type (input/output):"; n_bits "Bit width (output):"; bin_pt "Binary point (output):"
      mask help:
      | This vector accumulator based on DSP48 slices and BRAMs is designed for wide accumulators (48 < output width <= 96).
      |
      | It outputs its previous accumulated vector after a new_acc pulse is received.
      |
      | The "Data IN" (din) value is used if "Data OK" (dok) is 1, otherwise a 0 value is accumulated instead.  This can be used, for example, to implement blanking without requiring external multiplexers.
      mask init:
      | set_param([gcb,'/outsize/Reinterpret'], 'arith_type', arith_type);
      mask TypeOptions arith_type: Signed  (2's comp) | Unsigned
  wide_bram_vacc1 : Subsystem  AncestorBlock=casper_library_accumulators/wide_bram_vacc  mask(wide_bram_vacc){vec_len=2048, arith_type=Unsigned, n_bits=52, bin_pt=34}
      mask prompts: vec_len "Vector length:"; arith_type "Arithmetic type (input/output):"; n_bits "Bit width (output):"; bin_pt "Binary point (output):"
      mask help:
      | This vector accumulator based on DSP48 slices and BRAMs is designed for wide accumulators (48 < output width <= 96).
      |
      | It outputs its previous accumulated vector after a new_acc pulse is received.
      |
      | The "Data IN" (din) value is used if "Data OK" (dok) is 1, otherwise a 0 value is accumulated instead.  This can be used, for example, to implement blanking without requiring external multiplexers.
      mask init:
      | set_param([gcb,'/outsize/Reinterpret'], 'arith_type', arith_type);
      mask TypeOptions arith_type: Signed  (2's comp) | Unsigned
  wide_bram_vacc2 : Subsystem  AncestorBlock=casper_library_accumulators/wide_bram_vacc  mask(wide_bram_vacc){vec_len=2048, arith_type=Unsigned, n_bits=52, bin_pt=34}
      mask prompts: vec_len "Vector length:"; arith_type "Arithmetic type (input/output):"; n_bits "Bit width (output):"; bin_pt "Binary point (output):"
      mask help:
      | This vector accumulator based on DSP48 slices and BRAMs is designed for wide accumulators (48 < output width <= 96).
      |
      | It outputs its previous accumulated vector after a new_acc pulse is received.
      |
      | The "Data IN" (din) value is used if "Data OK" (dok) is 1, otherwise a 0 value is accumulated instead.  This can be used, for example, to implement blanking without requiring external multiplexers.
      mask init:
      | set_param([gcb,'/outsize/Reinterpret'], 'arith_type', arith_type);
      mask TypeOptions arith_type: Signed  (2's comp) | Unsigned
  wide_bram_vacc3 : Subsystem  AncestorBlock=casper_library_accumulators/wide_bram_vacc  mask(wide_bram_vacc){vec_len=2048, arith_type=Unsigned, n_bits=52, bin_pt=34}
      mask prompts: vec_len "Vector length:"; arith_type "Arithmetic type (input/output):"; n_bits "Bit width (output):"; bin_pt "Binary point (output):"
      mask help:
      | This vector accumulator based on DSP48 slices and BRAMs is designed for wide accumulators (48 < output width <= 96).
      |
      | It outputs its previous accumulated vector after a new_acc pulse is received.
      |
      | The "Data IN" (din) value is used if "Data OK" (dok) is 1, otherwise a 0 value is accumulated instead.  This can be used, for example, to implement blanking without requiring external multiplexers.
      mask init:
      | set_param([gcb,'/outsize/Reinterpret'], 'arith_type', arith_type);
      mask TypeOptions arith_type: Signed  (2's comp) | Unsigned
  wide_bram_vacc4 : Subsystem  AncestorBlock=casper_library_accumulators/wide_bram_vacc  mask(wide_bram_vacc){vec_len=2048, arith_type=Unsigned, n_bits=52, bin_pt=34}
      mask prompts: vec_len "Vector length:"; arith_type "Arithmetic type (input/output):"; n_bits "Bit width (output):"; bin_pt "Binary point (output):"
      mask help:
      | This vector accumulator based on DSP48 slices and BRAMs is designed for wide accumulators (48 < output width <= 96).
      |
      | It outputs its previous accumulated vector after a new_acc pulse is received.
      |
      | The "Data IN" (din) value is used if "Data OK" (dok) is 1, otherwise a 0 value is accumulated instead.  This can be used, for example, to implement blanking without requiring external multiplexers.
      mask init:
      | set_param([gcb,'/outsize/Reinterpret'], 'arith_type', arith_type);
      mask TypeOptions arith_type: Signed  (2's comp) | Unsigned
  wide_bram_vacc5 : Subsystem  AncestorBlock=casper_library_accumulators/wide_bram_vacc  mask(wide_bram_vacc){vec_len=2048, arith_type=Unsigned, n_bits=52, bin_pt=34}
      mask prompts: vec_len "Vector length:"; arith_type "Arithmetic type (input/output):"; n_bits "Bit width (output):"; bin_pt "Binary point (output):"
      mask help:
      | This vector accumulator based on DSP48 slices and BRAMs is designed for wide accumulators (48 < output width <= 96).
      |
      | It outputs its previous accumulated vector after a new_acc pulse is received.
      |
      | The "Data IN" (din) value is used if "Data OK" (dok) is 1, otherwise a 0 value is accumulated instead.  This can be used, for example, to implement blanking without requiring external multiplexers.
      mask init:
      | set_param([gcb,'/outsize/Reinterpret'], 'arith_type', arith_type);
      mask TypeOptions arith_type: Signed  (2's comp) | Unsigned
  wide_bram_vacc6 : Subsystem  AncestorBlock=casper_library_accumulators/wide_bram_vacc  mask(wide_bram_vacc){vec_len=2048, arith_type=Unsigned, n_bits=52, bin_pt=34}
      mask prompts: vec_len "Vector length:"; arith_type "Arithmetic type (input/output):"; n_bits "Bit width (output):"; bin_pt "Binary point (output):"
      mask help:
      | This vector accumulator based on DSP48 slices and BRAMs is designed for wide accumulators (48 < output width <= 96).
      |
      | It outputs its previous accumulated vector after a new_acc pulse is received.
      |
      | The "Data IN" (din) value is used if "Data OK" (dok) is 1, otherwise a 0 value is accumulated instead.  This can be used, for example, to implement blanking without requiring external multiplexers.
      mask init:
      | set_param([gcb,'/outsize/Reinterpret'], 'arith_type', arith_type);
      mask TypeOptions arith_type: Signed  (2's comp) | Unsigned
  wide_bram_vacc7 : Subsystem  AncestorBlock=casper_library_accumulators/wide_bram_vacc  mask(wide_bram_vacc){vec_len=2048, arith_type=Unsigned, n_bits=52, bin_pt=34}
      mask prompts: vec_len "Vector length:"; arith_type "Arithmetic type (input/output):"; n_bits "Bit width (output):"; bin_pt "Binary point (output):"
      mask help:
      | This vector accumulator based on DSP48 slices and BRAMs is designed for wide accumulators (48 < output width <= 96).
      |
      | It outputs its previous accumulated vector after a new_acc pulse is received.
      |
      | The "Data IN" (din) value is used if "Data OK" (dok) is 1, otherwise a 0 value is accumulated instead.  This can be used, for example, to implement blanking without requiring external multiplexers.
      mask init:
      | set_param([gcb,'/outsize/Reinterpret'], 'arith_type', arith_type);
      mask TypeOptions arith_type: Signed  (2's comp) | Unsigned
  data_valid : Outport
  power0 : Outport  Port=2
  power1 : Outport  Port=3
  power2 : Outport  Port=4
  power3 : Outport  Port=5
  power4 : Outport  Port=6
  power5 : Outport  Port=7
  power6 : Outport  Port=8
  power7 : Outport  Port=9
  wires:
  Slice6/1 -> power0/1
  Slice8/1 -> power1/1
  sync/1 -> new_acc1/1(sync)
  Reinterpret1/1 -> Slice6/1
  Reinterpret4/1 -> Slice8/1
  wide_bram_vacc1/2(valid) -> Terminator24/1
  Reinterpret2/1 -> Slice1/1
  wide_bram_vacc2/2(valid) -> Terminator1/1
  Slice1/1 -> power2/1
  Slice3/1 -> power3/1
  Reinterpret5/1 -> Slice3/1
  wide_bram_vacc3/2(valid) -> Terminator3/1
  Reinterpret3/1 -> Slice2/1
  wide_bram_vacc4/2(valid) -> Terminator2/1
  Slice2/1 -> power4/1
  Reinterpret6/1 -> Slice4/1
  wide_bram_vacc5/2(valid) -> Terminator4/1
  Slice4/1 -> power5/1
  Slice7/1 -> power6/1
  Reinterpret8/1 -> Slice7/1
  Reinterpret7/1 -> Slice5/1
  Slice5/1 -> power7/1
  wide_bram_vacc6/2(valid) -> Terminator6/1
  wide_bram_vacc7/2(valid) -> Terminator5/1
  acc_length/1 -> new_acc1/2(acc_len)
  acc_start_skip/1 -> new_acc1/3(acc_start_skip)
  new_acc1/2(use_data) -> Delay34/1
  [use_data] -> Delay2/1
  new_acc1/1(new_acc) -> Delay33/1
  [new_acc] -> Delay19/1
  [use_data] -> Delay23/1
  [new_acc] -> Delay24/1
  [use_data] -> Delay21/1
  [new_acc] -> Delay22/1
  [use_data] -> Delay18/1
  [new_acc] -> Delay20/1
  [use_data] -> Delay16/1
  [new_acc] -> Delay17/1
  [use_data] -> Delay14/1
  [new_acc] -> Delay15/1
  [use_data] -> Delay12/1
  [new_acc] -> Delay13/1
  [use_data] -> Delay11/1
  [new_acc] -> Delay10/1
  power_in0/1 -> Delay25/1
  power_in1/1 -> Delay26/1
  power_in2/1 -> Delay27/1
  power_in3/1 -> Delay28/1
  power_in4/1 -> Delay29/1
  power_in5/1 -> Delay30/1
  power_in6/1 -> Delay31/1
  power_in7/1 -> Delay32/1
  wide_bram_vacc7/1(dout) -> Reinterpret7/1
  wide_bram_vacc6/1(dout) -> Reinterpret8/1
  wide_bram_vacc5/1(dout) -> Reinterpret6/1
  wide_bram_vacc4/1(dout) -> Reinterpret3/1
  wide_bram_vacc3/1(dout) -> Reinterpret5/1
  wide_bram_vacc2/1(dout) -> Reinterpret2/1
  wide_bram_vacc1/1(dout) -> Reinterpret4/1
  wide_bram_vacc/1(dout) -> Reinterpret1/1
  wide_bram_vacc/2(valid) -> data_valid/1
  Delay19/1 -> wide_bram_vacc/1(new_acc)
  Delay1/1 -> wide_bram_vacc/2(din)
  Delay2/1 -> wide_bram_vacc/3(dok)
  Delay3/1 -> wide_bram_vacc1/2(din)
  Delay4/1 -> wide_bram_vacc2/2(din)
  Delay5/1 -> wide_bram_vacc3/2(din)
  Delay6/1 -> wide_bram_vacc4/2(din)
  Delay7/1 -> wide_bram_vacc5/2(din)
  Delay8/1 -> wide_bram_vacc6/2(din)
  Delay9/1 -> wide_bram_vacc7/2(din)
  Delay10/1 -> wide_bram_vacc7/1(new_acc)
  Delay11/1 -> wide_bram_vacc7/3(dok)
  Delay12/1 -> wide_bram_vacc6/3(dok)
  Delay13/1 -> wide_bram_vacc6/1(new_acc)
  Delay14/1 -> wide_bram_vacc5/3(dok)
  Delay15/1 -> wide_bram_vacc5/1(new_acc)
  Delay16/1 -> wide_bram_vacc4/3(dok)
  Delay17/1 -> wide_bram_vacc4/1(new_acc)
  Delay18/1 -> wide_bram_vacc3/3(dok)
  Delay20/1 -> wide_bram_vacc3/1(new_acc)
  Delay21/1 -> wide_bram_vacc2/3(dok)
  Delay22/1 -> wide_bram_vacc2/1(new_acc)
  Delay23/1 -> wide_bram_vacc1/3(dok)
  Delay24/1 -> wide_bram_vacc1/1(new_acc)
  Delay25/1 -> Delay35/1
  Delay26/1 -> Delay36/1
  Delay27/1 -> Delay37/1
  Delay28/1 -> Delay38/1
  Delay29/1 -> Delay39/1
  Delay30/1 -> Delay40/1
  Delay31/1 -> Delay41/1
  Delay32/1 -> Delay42/1
  Delay33/1 -> [new_acc]
  Delay34/1 -> [use_data]
  Delay35/1 -> Delay1/1
  Delay36/1 -> Delay3/1
  Delay37/1 -> Delay4/1
  Delay38/1 -> Delay5/1
  Delay39/1 -> Delay6/1
  Delay40/1 -> Delay7/1
  Delay41/1 -> Delay8/1
  Delay42/1 -> Delay9/1
